simulink model "EstimadorFriccionB"  (R2015a)
settings: Solver=ode45  StartTime=0.0  StopTime=40  RelTol=1e-3
libraries: simulink x1, cstblocks x1
settings Model: Creator=Usuario  LastModifiedBy=Usuario

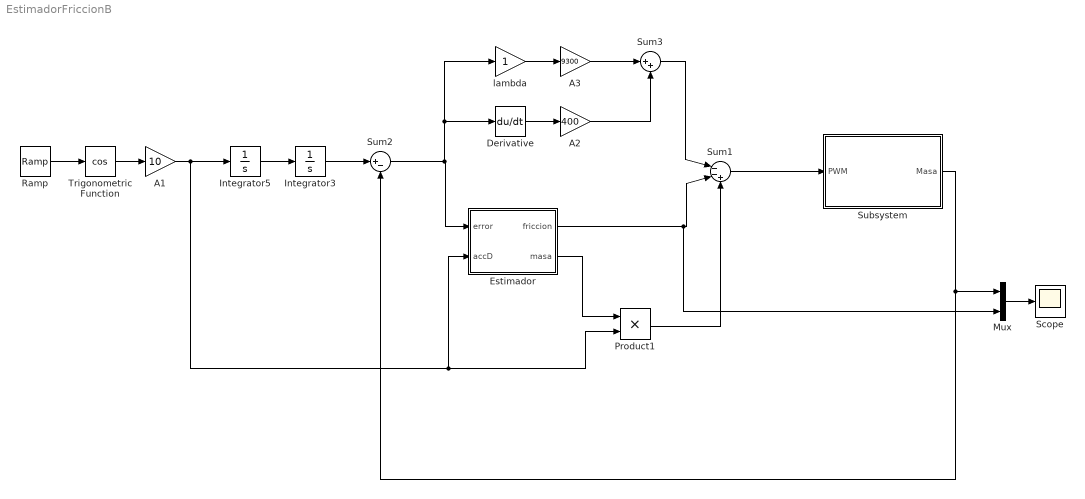
== system EstimadorFriccionB ==
  A1 : Gain  Gain=10
  A2 : Gain  Gain=400
  A3 : Gain  Gain=9300
  Derivative : Derivative
  Estimador : Subsystem
  Integrator3 : Integrator
  Integrator5 : Integrator
  Mux : Mux  Inputs=2
  Product1 : Product
  Ramp : simulink/Sources/Ramp  slope=0.1  start=0  X0=0
  Scope : Scope
      settings: TimeRange=10  YMin=0  YMax=2
  Subsystem : Subsystem
  Sum1 : Sum  Inputs=|--+
  Sum2 : Sum  Inputs=|+-
  Sum3 : Sum  Inputs=|++
  Trigonometric Function : Trigonometry  Operator=cos
  lambda : Gain
  wires:
  Integrator5/1 -> Integrator3/1
  Trigonometric Function/1 -> A1/1
  Mux/1 -> Scope/1
  Ramp/1 -> Trigonometric Function/1
  A1/1 -> Estimador/2(accD), Product1/2, Integrator5/1
  Subsystem/1(Masa) -> Mux/1, Sum2/2
  Sum1/1 -> Subsystem/1(PWM)
  Estimador/2(masa) -> Product1/1
  Estimador/1(friccion) -> Mux/2, Sum1/2
  Product1/1 -> Sum1/3
  Integrator3/1 -> Sum2/1
  Sum2/1 -> lambda/1, Derivative/1, Estimador/1(error)
  Derivative/1 -> A2/1
  A3/1 -> Sum3/1
  A2/1 -> Sum3/2
  Sum3/1 -> Sum1/1
  lambda/1 -> A3/1

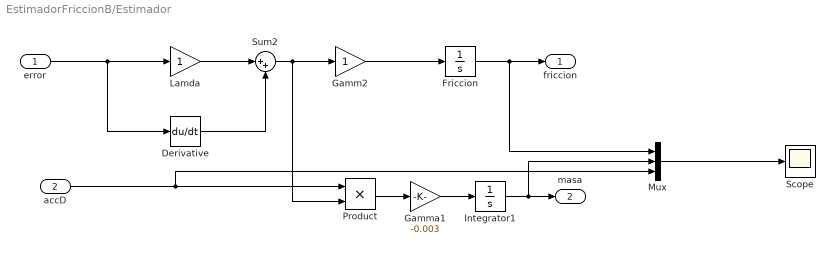
== system EstimadorFriccionB/Estimador ==
  error : Inport
  accD : Inport  Port=2
  Derivative : Derivative
  Friccion : Integrator  InitialCondition=-0.2
  Gamm2 : Gain
  Gamma1 : Gain  Gain=-0.003
  Integrator1 : Integrator  InitialCondition=5.7
  Lamda : Gain
  Mux : Mux  Inputs=3
  Product : Product
  Scope : Scope
  Sum2 : Sum  Inputs=|++
  friccion : Outport
  masa : Outport  Port=2
  wires:
  error/1 -> Derivative/1, Lamda/1
  Lamda/1 -> Sum2/1
  Derivative/1 -> Sum2/2
  Sum2/1 -> Product/2, Gamm2/1
  Gamm2/1 -> Friccion/1
  accD/1 -> Mux/3, Product/1
  Gamma1/1 -> Integrator1/1
  Product/1 -> Gamma1/1
  Integrator1/1 -> Mux/2, masa/1
  Friccion/1 -> Mux/1, friccion/1
  Mux/1 -> Scope/1

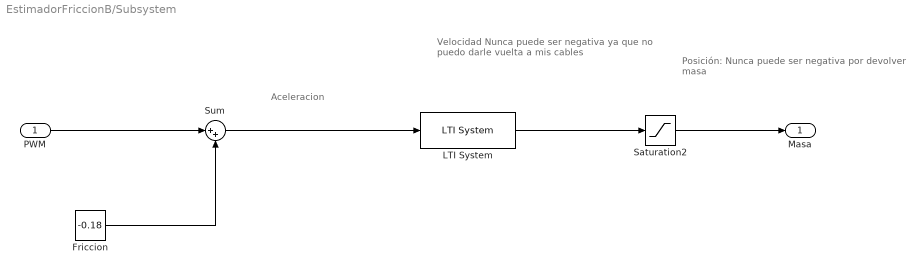
== system EstimadorFriccionB/Subsystem ==
  note: Posición:
      | Nunca puede ser negativa por devolver masa
  note: Velocidad
      | Nunca puede ser negativa ya que no puedo
      | darle vuelta a mis cables
  note: Aceleracion
  PWM : Inport
  Friccion : Constant  Value=-0.18
  LTI System : cstblocks/LTI System  sys=Gs  IC=[]
  Saturation2 : Saturate  UpperLimit=100000  LowerLimit=0
  Sum : Sum  Inputs=|++
  Masa : Outport
  wires:
  PWM/1 -> Sum/1
  Friccion/1 -> Sum/2
  LTI System/1 -> Saturation2/1
  Sum/1 -> LTI System/1
  Saturation2/1 -> Masa/1
